simulink model "AnhKhoa_Controller"  (R2020b)
settings: Solver=VariableStepAuto  StartTime=0.0  StopTime=100  RelTol=1e-3
values from neighbouring files (symbols this model uses):
  A_AD = horzcat(A_i, A_ii)    [Trial_Script.m]    (also in mpc_misoo.m)
  B_AD = horzcat(B_i, B_ii)    [Trial_Script.m]    (also in mpc_misoo.m)
  C_AD = eye(6)    [Trial_Script.m]    (also in mpc_misoo.m)
  C_D = 0.6    [Trial_Script.m]
  D_AD = zeros(6)    [Trial_Script.m]    (also in mpc_misoo.m)
  rho = 1.225    [Trial_Script.m]
  S = 1*1.8    (= 1.8)    [Trial_Script.m]
  T = 10.5    [Trial_Script.m]    (also in temp2.m = readtable('proparms.txt','Delimiter',' '))
  v_vehicle = [20; 0; 0]    [Trial_Script.m]
  x_cp = [0.3; 0.2; 0.1]    [Trial_Script.m]
libraries: mpclib x1, cstblocks x1
settings Model: Creator=Jonathan van Zyl  LastModifiedBy=Jonathan van Zyl

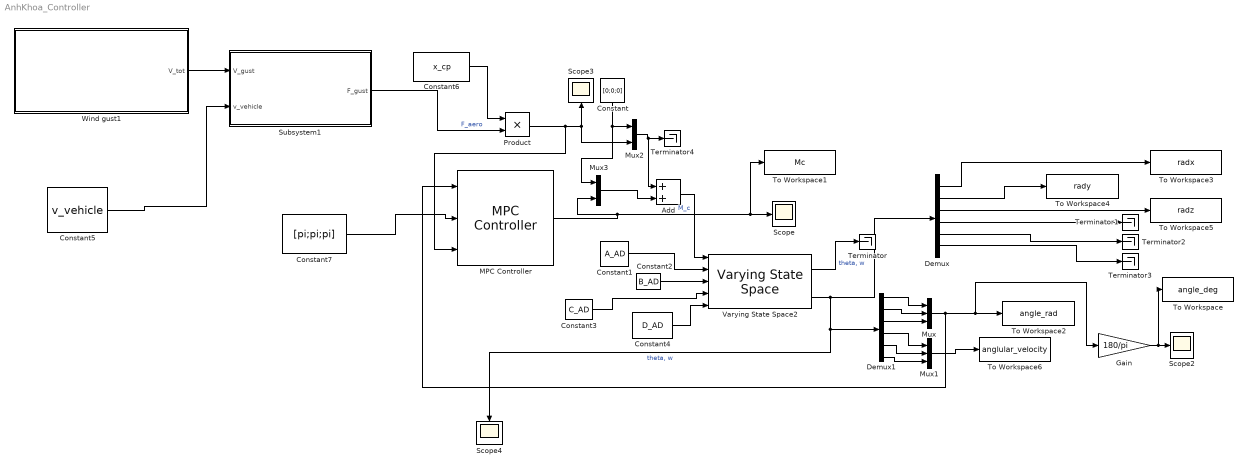
== system AnhKhoa_Controller ==
  Add : Sum
  Constant : Constant  Value=[0;0;0]
  Constant1 : Constant  Value=A_AD
  Constant2 : Constant  Value=B_AD
  Constant3 : Constant  Value=C_AD
  Constant4 : Constant  Value=D_AD
  Constant5 : Constant  Value=v_vehicle
  Constant6 : Constant  Value=x_cp
  Constant7 : Constant  Value=[pi;pi;pi]
  Demux : Demux  Outputs=6
  Demux1 : Demux  Outputs=6
  Gain : Gain  Gain=180/pi
  MPC Controller : mpclib/MPC Controller  SCDEnableBlockLinearizationSpecification=on  mpcobj=mpc1  is_multiple=0  enable_value=0  return_u0=off  updateMPCinCallerWorkspace=on  md_inport=on  mv_inport=off  uref_inport=off  return_cost=off  return_mvseq=off  return_qpstatus=off  return_xseq=off  return_state=off  return_ovseq=off  state_inport=off  umin_inport=off  umax_inport=off  ymin_inport=off  ymax_inport=off  cc_inport=off  ywt_inport=off  uwt_inport=off  duwt_inport=off  rhoeps_inport=off  pm_inport=off  MaximumP=10  HorizonChoice=FixedHorizon  n_ts=1  n_p=10  n_mv=3  n_md=3  n_ud=0  n_mo=3  n_uo=0  BlockDataType=double  SampleTimeInherited=off  switch_inport=off
  Mux : Mux  Inputs=3
  Mux1 : Mux  Inputs=3
  Mux2 : Mux  Inputs=2
  Mux3 : Mux  Inputs=2
  Product : Product
  Scope{,2..4} (4 alike) : Scope
  Subsystem1 : Subsystem
  Terminator{,1..4} (5 alike) : Terminator
  To Workspace : ToWorkspace  VariableName=angle_deg  SaveFormat=Timeseries  SampleTime=-1
  To Workspace1 : ToWorkspace  VariableName=Mc  SaveFormat=Timeseries  SampleTime=-1
      settings: Save2DSignal=2-D array (concatenate along first dimension)
  To Workspace2 : ToWorkspace  VariableName=angle_rad  SaveFormat=Timeseries  SampleTime=-1
  To Workspace3 : ToWorkspace  VariableName=radx  SaveFormat=Timeseries  SampleTime=-1
  To Workspace4 : ToWorkspace  VariableName=rady  SaveFormat=Timeseries  SampleTime=-1
  To Workspace5 : ToWorkspace  VariableName=radz  SaveFormat=Timeseries  SampleTime=-1
  To Workspace6 : ToWorkspace  VariableName=anglular_velocity  SaveFormat=Timeseries  SampleTime=-1
  Varying State Space2 : cstblocks/Linear Parameter Varying/Varying State Space  x0=0  xNames=''  OutputX=on  OutputDX=off
  Wind gust1 : Subsystem
  wires:
  Constant5/1 -> Subsystem1/2(v_vehicle)
  Demux/1 -> To Workspace3/1
  Demux/2 -> To Workspace4/1
  Gain/1 -> To Workspace/1, Scope2/1
  Subsystem1/1(F_gust) -> Product/2  "F_aero"
  Constant6/1 -> Product/1
  Wind gust1/1(V_tot) -> Subsystem1/1(V_gust)
  Product/1 -> MPC Controller/3, Mux2/2, Scope3/1
  Constant1/1 -> Varying State Space2/2
  Constant4/1 -> Varying State Space2/5
  Varying State Space2/2 -> Demux1/1, Scope4/1, Demux/1  "theta, w"
  MPC Controller/1 -> Mux3/2, To Workspace1/1, Scope/1  "M_c"
  Varying State Space2/1 -> Terminator/1  "theta, w"
  Constant2/1 -> Varying State Space2/3
  Mux3/1 -> Add/2
  Constant3/1 -> Varying State Space2/4
  Demux/3 -> To Workspace5/1
  Constant7/1 -> MPC Controller/2
  Demux/4 -> Terminator1/1
  Demux/5 -> Terminator2/1
  Demux/6 -> Terminator3/1
  Demux1/1 -> Mux/1
  Mux/1 -> MPC Controller/1, Gain/1, To Workspace2/1
  Demux1/2 -> Mux/2
  Demux1/3 -> Mux/3
  Demux1/4 -> Mux1/1
  Demux1/5 -> Mux1/2
  Demux1/6 -> Mux1/3
  Mux1/1 -> To Workspace6/1
  Constant/1 -> Mux3/1, Mux2/1
  Mux2/1 -> Add/1, Terminator4/1
  Add/1 -> Varying State Space2/1

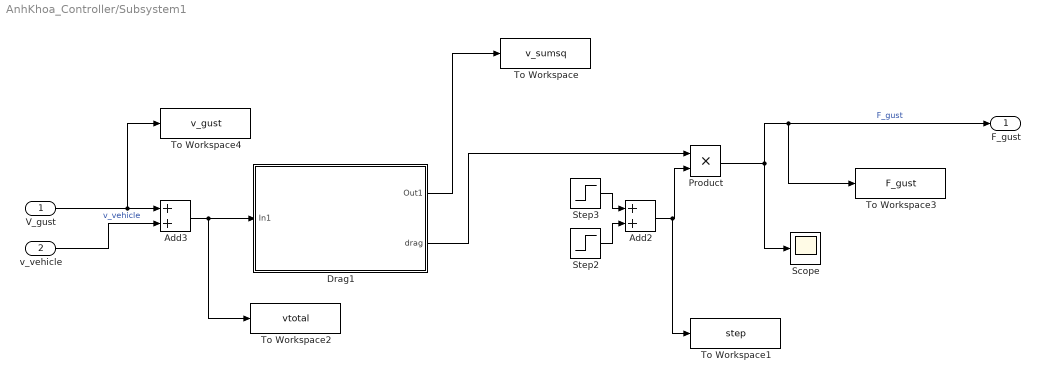
== system AnhKhoa_Controller/Subsystem1 ==
  V_gust : Inport
  v_vehicle : Inport  Port=2
  Add2 : Sum
  Add3 : Sum
  Drag1 : Subsystem
  Product : Product
  Scope : Scope
  Step2 : Step  Time=0  SampleTime=0
  Step3 : Step  Time=10.5  After=-1  SampleTime=0
  To Workspace : ToWorkspace  VariableName=v_sumsq  SampleTime=-1
  To Workspace1 : ToWorkspace  VariableName=step  SaveFormat=Timeseries  SampleTime=-1
  To Workspace2 : ToWorkspace  VariableName=vtotal  SaveFormat=Timeseries  SampleTime=-1
  To Workspace3 : ToWorkspace  VariableName=F_gust  SaveFormat=Timeseries  SampleTime=-1
  To Workspace4 : ToWorkspace  VariableName=v_gust  SaveFormat=Timeseries  SampleTime=-1
  F_gust : Outport
  wires:
  Product/1 -> F_gust/1, To Workspace3/1, Scope/1  "F_gust"
  Step3/1 -> Add2/1
  V_gust/1 -> To Workspace4/1, Add3/1
  Drag1/1(Out1) -> To Workspace/1
  Add3/1 -> Drag1/1(In1), To Workspace2/1
  Add2/1 -> To Workspace1/1, Product/2
  Step2/1 -> Add2/2
  v_vehicle/1 -> Add3/2  "v_vehicle"
  Drag1/2(drag) -> Product/1

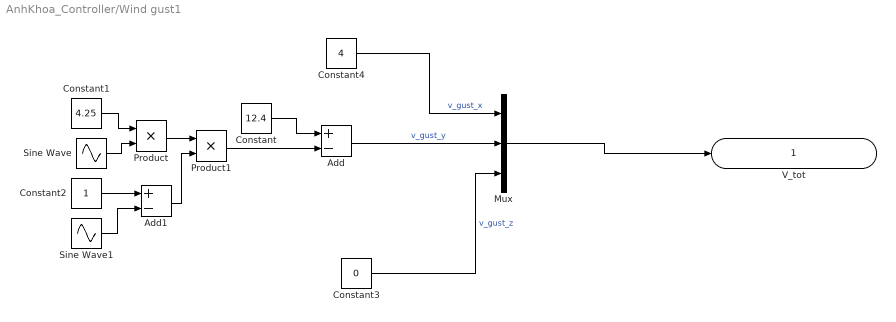
== system AnhKhoa_Controller/Wind gust1 ==
  Add : Sum  Inputs=+-
  Add1 : Sum  Inputs=+-
  Constant : Constant  Value=12.4
  Constant1 : Constant  Value=4.25
  Constant2 : Constant
  Constant3 : Constant  Value=0
  Constant4 : Constant  Value=4  VectorParams1D=off
  Mux : Mux  Inputs=3
  Product : Product
  Product1 : Product
  Sine Wave : Sin  Frequency=3*pi/T  SampleTime=0
  Sine Wave1 : Sin  Frequency=2*pi/T  Phase=pi/2  SampleTime=0
  V_tot : Outport
  wires:
  Constant/1 -> Add/1
  Constant1/1 -> Product/1
  Sine Wave/1 -> Product/2
  Constant2/1 -> Add1/1
  Sine Wave1/1 -> Add1/2
  Product/1 -> Product1/1
  Add1/1 -> Product1/2
  Product1/1 -> Add/2
  Add/1 -> Mux/2  "v_gust_y"
  Constant3/1 -> Mux/3  "v_gust_z"
  Mux/1 -> V_tot/1
  Constant4/1 -> Mux/1  "v_gust_x"

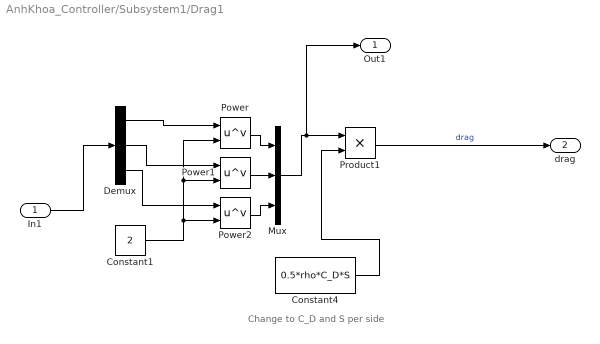
== system AnhKhoa_Controller/Subsystem1/Drag1 ==
  note: Change to C_D and S per side
  In1 : Inport
  Constant1 : Constant  Value=2
  Constant4 : Constant  Value=0.5*rho*C_D*S
  Demux : Demux  Outputs=3
  Mux : Mux  Inputs=3
  Power : Math  Operator=pow  SaturateOnIntegerOverflow=on
  Power1 : Math  Operator=pow  SaturateOnIntegerOverflow=on
  Power2 : Math  Operator=pow  SaturateOnIntegerOverflow=on
  Product1 : Product
  Out1 : Outport
  drag : Outport  Port=2
  wires:
  Constant1/1 -> Power2/2, Power1/2, Power/2
  Power2/1 -> Mux/3
  Power/1 -> Mux/1
  In1/1 -> Demux/1
  Demux/1 -> Power/1
  Demux/3 -> Power2/1
  Demux/2 -> Power1/1
  Power1/1 -> Mux/2
  Constant4/1 -> Product1/2
  Mux/1 -> Out1/1, Product1/1
  Product1/1 -> drag/1  "drag"
